simulink model "KalmanBlock"  (Simulink 5.0)
settings: Solver=ode45  StartTime=0.0  StopTime=0.1  RelTol=1e-3
settings Model: LastModifiedBy=Praveen

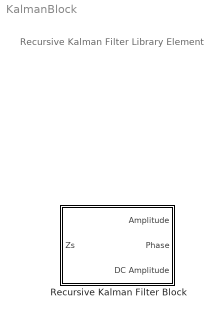
== system KalmanBlock ==
  note: Recursive Kalman Filter Library Element
  Recursive Kalman Filter Block : Subsystem  mask(Kalman Block){f=60, Fs=32, X0=[0;0;0], C=[1 0 1], sigman=0.01, sigmav=0.005, M=[(0.24^2) 0 0;0 (0.24^2) 0;0 0 (0.24^2)], lambda=1000}
      mask prompts: f "Fundamental Frequency of Input Signal (f) in Hz"; Fs "Sampling Frequency (Fs) in samples per second"; X0 "Initial State (x0)"; C "Voltage-Phasor relation matrix (C)"; sigman "Measurement Noise Variance (Sigma n)"; sigmav "Process noise variance (Sigma v)"; M "Single step transition error covariance (M)"; lambda "Decaying DC Parameter (lambda)"
      mask help:
      | Measures the Phasor voltage values using the Kalman filter.
      | The input to the block is 'Zs(n)', the signal at time nT. 'f' is the fundamental frequency of the signal, and the harmonics are assumed to be integral multiple of this.
      | 'C' is the ralationship between voltage and phasor values. The default value is [1,0,1] assuming zero imaginary component and non-zero DC component.
      | Measurement noise variance 'sigman' models the noise during the voltage measurement.
      | Process variance 'sigmav' denotes the variation in the measurement of voltage values.
      | 'M' denotes the single step variation
      | Decaying DC component models the decreasing nature of the DC.

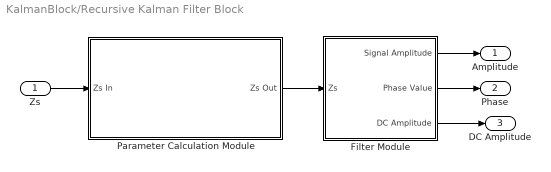
== system KalmanBlock/Recursive Kalman Filter Block ==
  Zs : Inport
  Filter Module : Subsystem  Priority=2
  Parameter Calculation Module : Subsystem  Priority=1
      mask Display:
      | disp('PARAMETER MODULE');
      | port_label('input',1,'Zs in');
      | port_label('output',1,'Zs out');
  Amplitude : Outport
  Phase : Outport  Port=2
  DC Amplitude : Outport  Port=3
  wires:
  Zs/1 -> Parameter Calculation Module/1(Zs In)
  Parameter Calculation Module/1(Zs Out) -> Filter Module/1(Zs)
  Filter Module/1(Signal Amplitude) -> Amplitude/1
  Filter Module/3(DC Amplitude) -> DC Amplitude/1
  Filter Module/2(Phase Value) -> Phase/1

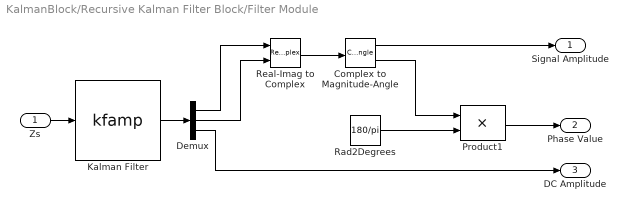
== system KalmanBlock/Recursive Kalman Filter Block/Filter Module ==
  Zs : Inport
  Complex to Magnitude-Angle : ComplexToMagnitudeAngle
  Demux : Demux  Outputs=3
  Kalman Filter : S-Function  Priority=2  FunctionName=kfamp  Parameters=X0 C M
      mask Type: Kalman Filter Block
  Product1 : Product  ShowAdditionalParam=on  SaturateOnIntegerOverflow=on
  Rad2Degrees : Constant  Value=180/pi
  Real-Imag to Complex : RealImagToComplex
  Signal Amplitude : Outport
  Phase Value : Outport  Port=2
  DC Amplitude : Outport  Port=3
  wires:
  Zs/1 -> Kalman Filter/1
  Kalman Filter/1 -> Demux/1
  Demux/1 -> Real-Imag to Complex/1
  Demux/2 -> Real-Imag to Complex/2
  Demux/3 -> DC Amplitude/1
  Product1/1 -> Phase Value/1
  Real-Imag to Complex/1 -> Complex to Magnitude-Angle/1
  Complex to Magnitude-Angle/1 -> Signal Amplitude/1
  Rad2Degrees/1 -> Product1/2
  Complex to Magnitude-Angle/2 -> Product1/1

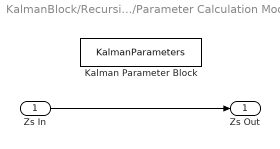
== system KalmanBlock/Recursive Kalman Filter Block/Parameter Calculation Module ==
  Zs In : Inport
  Kalman Parameter Block : S-Function  Priority=1  FunctionName=KalmanParameters  Parameters=Fs f sigman sigmav M lambda
  Zs Out : Outport
  wires:
  Zs In/1 -> Zs Out/1
